simulink library "HMMtoolbox"  (Simulink 8.3)
settings: Solver=ode45  StartTime=0.0  StopTime=10.0  RelTol=1e-3
undefined symbols (not defined in the file): HMMS
libraries: simulink x12
settings Model: Creator=Esrod Zuch  LastModifiedBy=shubo

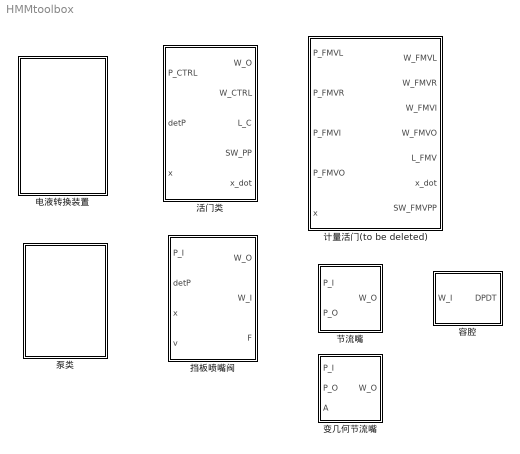
== system HMMtoolbox ==
  变几何节流嘴 : Subsystem  mask{Cqmax=HMMS.JLZ.Cq_max, lamc=1000, rho=HMMS.RHO, nu=HMMS.NU}
      mask prompts: Cqmax "Cq_max(最大流量系数)"; lamc "lamc(临界流数)"; rho "RHO(油液密度kg/m^3)"; nu "NU(油液运动粘度cP)"
  容腔 : Subsystem  mask{B=HMMS.B, V0=HMMS.V(2)}
      mask prompts: B "B(容腔模量kPa)"; V0 "V0(容腔体积m^3)"
  挡板喷嘴阀 : Subsystem  mask{rho=HMMS.RHO, Kv=HMMS.DBPZF.Kv, D_F=HMMS.DBPZF.D_F, D_I=HMMS.DBPZF.D_I, D_R=HMMS.DBPZF.D_R, mode_direct=相反, L_L=0, L_H=HMMS.DBPZF.L_H, x0=HMMS.DBPZF.x0}
      mask prompts: rho "RHO(油液密度kg/m^3)"; Kv "Kv(流量系数)"; D_F "挡板直径(mm)"; D_I "喷嘴内径(mm)"; D_R "杆径(mm)"; mode_direct "开度正方向与阀芯运动正方向"; L_L "L_L(开度低限mm)"; L_H "L_H(开度高限mm)"; x0 "x0(初始遮蔽量mm)"
      mask TypeOptions mode_direct: 相同 | 相反
  泵类 : Subsystem
  活门类 : Subsystem  mask{rho=HMMS.RHO, Kv=HMMS.LJHM.Kv, nu=51, lamc=100, D_P=HMMS.LJHM.D_P, D_R=[0 0], direct_CTRL=[1 -1], mode_direct=相同, L_L=0, L_H=HMMS.LJHM.L_H, m=HMMS.LJHM.m, k=HMMS.LJHM.k, f=HMMS.LJHM.f, f0=HMMS.LJHM.f0, x0=HMMS.LJHM.x0, mode_hole=插值表, C_I=HMMS.LJHM.C_I, C_O=HMMS.LJHM.C_O, D_HOLE=1, n=1}
      mask prompts: rho "RHO(油液密度kg/m^3)"; Kv "Kv_max(最大流量系数)"; nu "NU(油液运动粘度cP)"; lamc "lamc(临界流数)"; D_P "D_P向量(各腔筒径mm)"; D_R "D_R向量(各腔杆径mm)"; direct_CTRL "各腔压力方向向量(推为1拉为-1)"; mode_direct "开度正方向与阀芯运动正方向"; L_L "L_L(位移低限mm)"; L_H "L_H(位移高限mm)"; m "m(阀芯质量kg)"; k "k(弹簧弹性模量N/m)"; f "f(阀芯阻尼N/(m/s))"; f0 "f0(弹簧预紧力N)"; x0 "x0(初始遮蔽量mm)"; mode_hole "计算模式"; C_I "C_I(特性插值输入)"; C_O "C_O(特性插值输出)"; D_HOLE "D_HOLE(圆孔直径mm)"; n "n(圆孔数量)"
      mask TypeOptions mode_direct: 相同 | 相反
      mask TypeOptions mode_hole: 插值表 | 圆面积公式
      mask DialogControl Container13_copy Prompt: 插值表
      mask DialogControl Container13 Prompt: 圆面积公式
  电液转换装置 : Subsystem
  节流嘴 : Subsystem  mask{Cqmax=HMMS.JLZ.Cq_max, lamc=1000, d=HMMS.JLZ.D, rho=HMMS.RHO, nu=HMMS.NU}
      mask prompts: Cqmax "Cq_max(最大流量系数)"; lamc "lamc(临界流数)"; d "D(圆孔直径mm)"; rho "RHO(油液密度kg/m^3)"; nu "NU(油液运动粘度cP)"
  计量活门(to be deleted) : Subsystem  mask(计量活门){L_FMVL=0, L_FMVH=HMMS.HYHM.L_H, D_FMVLP=HMMS.HYHM.D_LP, D_FMVLR=0, D_FMVRP=HMMS.HYHM.D_RP, D_FMVRR=0, C_FMVI=HMMS.HYHM.C_I, C_FMVO=HMMS.HYHM.C_O, f0=HMMS.HYHM.f0, m_FMV=HMMS.HYHM.m, f_FMV=HMMS.HYHM.f, k=HMMS.HYHM.k, rho=HMMS.RHO, Kv_FMV=HMMS.HYHM.Kv}
      mask prompts: L_FMVL "L_FMVL(计量活门位移低限mm)"; L_FMVH "L_FMVH(计量活门位移高限mm)"; D_FMVLP "D_FMVLP(计量活门左腔筒径mm)"; D_FMVLR "D_FMVLR(计量活门左腔杆径mm)"; D_FMVRP "D_FMVRP(计量活门右腔筒径mm)"; D_FMVRR "D_FMVRR(计量活门右腔杆径mm)"; C_FMVI "C_FMVI(计量活门特性插值输入)"; C_FMVO "C_FMVO(计量活门特性插值输出)"; f0 "f0(弹簧预紧力N)"; m_FMV "m_FMV(计量活门阀芯质量kg)"; f_FMV "f_FMV(计量活门阀芯阻尼N/(m/s))"; k "k(计量活门弹簧弹性模量N/m)"; rho "ρ(油液密度kg/m^3)"; Kv_FMV "Kv_FMV(计量活门流量系数)"
      mask help: 填入相关参数

== system HMMtoolbox/变几何节流嘴 ==
  note: Cq
  note: kPa
  note: d/m
  note: m**2/s
  note: Cqmax
  note: m**2
  P_I : Inport
  P_O : Inport  Port=2
  A : Inport  Port=3
  Abs : Abs
  Add : Sum  Inputs=+-
  Constant : Constant  Value=Cqmax
  Constant6 : Constant  Value=nu
  Divide2 : Product  Inputs=*/
  Divide3 : Product  Inputs=**
  Divide4 : Product  Inputs=**
  Fcn : Fcn  Expr=sqrt(2*u*rho)
  Fcn1 : Fcn  Expr=sqrt(4*u/pi)
  Fcn2 : Fcn  Expr=tanh(2*u/lamc)
  Fcn3 : Fcn  Expr=u*1e-3/rho
  Gain1 : Gain  Gain=1e3
  Product : Product
  Product1 : Product  Inputs=3
  Sign : Signum  ZeroCross=off
  W_O : Outport
  wires:
  Sign/1 -> Product/2
  Fcn1/1 -> Divide2/1
  Product/1 -> W_O/1
  Fcn3/1 -> Divide2/2
  Constant6/1 -> Fcn3/1
  Add/1 -> Gain1/1
  Divide4/1 -> Product1/1
  Constant/1 -> Divide4/1
  Fcn2/1 -> Divide4/2
  Divide3/1 -> Fcn2/1
  Divide2/1 -> Divide3/1
  A/1 -> Fcn1/1, Product1/2
  P_I/1 -> Add/1
  Fcn/1 -> Product1/3, Divide3/2
  Abs/1 -> Fcn/1
  Product1/1 -> Product/1
  Gain1/1 -> Abs/1, Sign/1
  P_O/1 -> Add/2

== system HMMtoolbox/容腔 ==
  note: kg
  note: kPa
  note: kg/s
  note: dp/dt kPa/s
  note: V0 m**3
  W_I : Inport
  Constant : Constant  Value=B
  Constant1 : Constant  Value=V0
  Divide : Product  Inputs=**
  Divide1 : Product  Inputs=*/
  Gain1 : Gain  Gain=HMMS.RHO
  Sum of Elements : Sum  Inputs=+
  DPDT : Outport
  wires:
  Divide/1 -> Divide1/1
  Sum of Elements/1 -> Divide/1
  Constant/1 -> Divide/2
  W_I/1 -> Sum of Elements/1
  Divide1/1 -> DPDT/1
  Gain1/1 -> Divide1/2
  Constant1/1 -> Gain1/1

== system HMMtoolbox/挡板喷嘴阀 ==
  P_I : Inport
  detP : Inport  Port=2
  x : Inport  Port=3
  v : Inport  Port=4
  Add1 : Sum
  Add3 : Sum  Inputs=+-
  Gain1 : Gain  Gain=pi*(D_I^2-D_R^2)*10^-3/4
  Gain2 : Gain  Gain=pi*(D_F^2-D_I^2)*10^-3/4
  flowcalc : Subsystem
  W_O : Outport
  W_I : Outport  Port=2
  F : Outport  Port=3
  wires:
  flowcalc/1(W_O) -> W_O/1
  detP/1 -> Add3/2, flowcalc/1(detP)
  x/1 -> flowcalc/2(x)
  flowcalc/2(W_I) -> W_I/1
  v/1 -> flowcalc/3(v)
  P_I/1 -> Gain1/1, Add3/1
  Add3/1 -> Gain2/1
  Gain2/1 -> Add1/2
  Gain1/1 -> Add1/1
  Add1/1 -> F/1

== system HMMtoolbox/泵类 ==
  CLB : Subsystem  mask{mode=平均计算模式, RHO=780, ETA_hym=1, etamode=eta=constant, ETA_V_const=1, ETA_V_tab1=[0 1000 10000], ETA_V_tab2=[1 0.9 0.8], displ=2.2e-7, z1=10, z2=10, m_CLB=2, alpha=20, b_CLB=6}
      mask prompts: mode "齿轮泵计算模式"; RHO "RHO(工质密度kg/m^3)"; ETA_hym "ETA_hym(水力机械效率)"; etamode "计算模式"; ETA_V_const "ETA_V_const(效率常数)"; ETA_V_tab1 "N_tab(转速表rpm)"; ETA_V_tab2 "ETA_V_tab(效率表)"; displ "displ(排量m^3/rad)"; z1 "z1(主动轮齿数(个))"; z2 "z2(从动轮齿数(个))"; m_CLB "m(齿轮模数mm)"; alpha "alpha(齿轮压力角(°))"; b_CLB "b(齿宽mm)"
      mask TypeOptions mode: 平均计算模式 | 脉动计算模式
      mask TypeOptions etamode: eta=constant | eta=f(n)
      mask DialogControl ParameterGroupVar Prompt: 齿轮泵参数设置
      mask DialogControl Container12 Prompt: 模式：eta=constant
      mask DialogControl Container13 Prompt: 模式：eta=f(n)
  LXB : Subsystem  mask{mode=f(qv), ETA=0.8, RHO=780, D=10, D_r=10, N_r=26230, RHO_r=780, W_tab_1=[10000 20000 30000 40000 46400]/780/3600, P_tab_1=[7640	7830	7860	7530	7110], N_tab_2=[18361 19673 20984 22296 23607 24919 26230], W_tab_2=[10000 20000 30000 40000 46400]/780/3600, P_tab_2=[4250,4310,3950,3760,3638.4;4590,4670,4480,4280,4152;5130,5250,5160,4750,4561.76;5680,5830,5740,5400,5200;6280,6430,6400,6050,5700;6970,7150,7140,6800,6430;7640,7830,7860,7530,7110;]}
      mask prompts: mode "mode(计算模式)"; ETA "ETA(泵的工作效率)"; RHO "RHO(实际工质密度(kg/m^3))"; D "D(泵的实际直径mm)"; D_r "D_r(泵的参考直径mm)"; N_r "N_r(泵的参考转速(r/min))"; RHO_r "RHO_r参考工质密度(kg/m^3)"; W_tab_1 "W_tab_1(流量表(m^3/s))"; P_tab_1 "P_tab_1(增压表kPa)"; N_tab_2 "N_tab_2(转速表(r/min))"; W_tab_2 "W_tab_2(流量表m^3/s)"; P_tab_2 "P_tab_2(增压表kPa)"
      mask help: 离心泵模型
      mask TypeOptions mode: f(qv) | f(qv,n)
      mask DialogControl Control2 Prompt: 离心泵模型
  ZSB : Subsystem  mask(柱塞泵){L_ZSBHX=15, D_ZSBZS=48*2, A_ZSBZS=23.8*23.8*pi/4, RHO=780, ETA_V=0.95, Z_ZSBZS=7, BETA_ZSBZS=11/180*pi, A_ZSBTJ=[pi*(33.26^2-17^2)/4, pi*(33.26^2-19.8^2)/4], L_ZSBTJ=[17*2.3/0.6,17*2.48/0.6,42.9,317.743165,165.3], k=((1421-754.6)/((139.7-101.9)-(139.7-119.6))+(1754-1313)/((158-96.8)-(158-114.6)))*1e3, BETA_ZSBSD=7/180*pi, L_x0=30+139.7, J_ZSBXP=0.34, KD=7.65}
      mask prompts: L_ZSBHX "L_HX(等效滑靴厚度mm)"; D_ZSBZS "D_ZS(柱塞轴线在缸体的分布圆直径mm)"; A_ZSBZS "A_ZS(柱塞截面面积mm^2)"; RHO "RHO(标准状态下，油液密度kg/m^3)"; ETA_V "ETA_V(容积效率)"; Z_ZSBZS "Z_ZS(柱塞数量)"; BETA_ZSBZS "BETA_ZS(柱塞安装角rad)"; A_ZSBTJ "A_TJ(面积参数向量mm^2)"; L_ZSBTJ "L_TJ(距离参数向量mm)"; k "k(弹簧弹性模量N/m)"; BETA_ZSBSD "BETA_SD(随动活塞安装角rad)"; L_x0 "L_x0(随动活塞初始位置mm)"; J_ZSBXP "J_XP(斜盘绕斜盘轴的转动惯量kg·m^2)"; KD "KD(斜盘转动阻力系数N·m·s/rad)"
      mask DialogControl DescTextVar Prompt: 填入相关参数

== system HMMtoolbox/活门类 ==
  P_CTRL : Inport
  detP : Inport  Port=2
  x : Inport  Port=3
  Constant4 : Constant  Value=0
  Demux : Demux  Outputs=2
  Gain5 : Gain  Gain=1000
  Mux : Mux  Inputs=2
  Mux1 : Mux  Inputs=2
  flowcalc : Subsystem
  motioncalc : Subsystem
  W_O : Outport
  W_CTRL : Outport  Port=2
  L_C : Outport  Port=3
  SW_PP : Outport  Port=4
  x_dot : Outport  Port=5
  wires:
  motioncalc/4(W_CTRL) -> W_CTRL/1
  flowcalc/1(W_O) -> W_O/1
  detP/1 -> flowcalc/1(detP)
  P_CTRL/1 -> motioncalc/1(P_CTRL)
  Gain5/1 -> L_C/1, flowcalc/2(L_C)
  Demux/2 -> motioncalc/2(v)  "velocity"
  x/1 -> Demux/1
  motioncalc/1(IsMoving) -> Mux1/2
  motioncalc/3(a) -> Mux/2
  Mux1/1 -> SW_PP/1
  Constant4/1 -> Mux1/1
  Demux/1 -> motioncalc/3(x), Gain5/1  "position"
  Mux/1 -> x_dot/1
  motioncalc/2(v_real) -> Mux/1

== system HMMtoolbox/电液转换装置 ==
  HSV23 : Subsystem  mask(电液伺服阀（单个孔特性验证）){Qm=HMMS.HSV23.W_R, delta_Pm=HMMS.HSV23.P_R, Im=HMMS.HSV23.I_R, Wn=HMMS.HSV23.Wn, ksi=HMMS.HSV23.XI, rho=HMMS.RHO}
      mask prompts: Qm "W_R(电液伺服阀额定流量kg/s)"; delta_Pm "P_R(电液伺服阀额定压降kPa)"; Im "I_R(额定电流mA)"; Wn "Wn(阀的自然频率rad/s)"; ksi "ξ(阀的阻尼比)"; rho "ρ(油液密度kg/m^3)"
      mask help: 填入相关参数，和AMESim数据一致
  HSV34 : Subsystem  mask(电液伺服阀（单个孔特性验证）){Qm=HMMS.HSV1.W_R, delta_Pm=HMMS.HSV1.P_R, Im=HMMS.HSV1.I_R, Idet=HMMS.HSV1.I_DELTA, Wn=HMMS.HSV1.Wn, ksi=HMMS.HSV1.XI, rho=HMMS.RHO}
      mask prompts: Qm "W_R(电液伺服阀额定流量kg/s)"; delta_Pm "P_R(电液伺服阀额定压降kPa)"; Im "I_R(额定电流mA)"; Idet "I_DELTA(电流偏置量mA)"; Wn "Wn(阀的自然频率rad/s)"; ksi "ξ(阀的阻尼比)"; rho "ρ(油液密度kg/m^3)"
      mask help: 填入相关参数，和AMESim数据一致

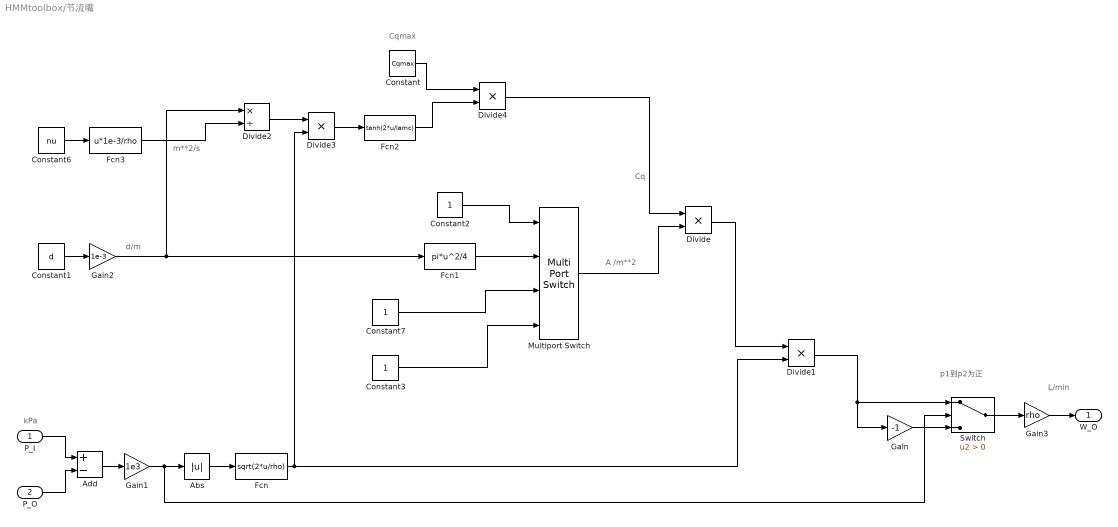
== system HMMtoolbox/节流嘴 ==
  note: L/min
  note: p1到p2为正
  note: Cqmax
  note: m**2/s
  note: d/m
  note: kPa
  note: A /m**2
  note: Cq
  P_I : Inport
  P_O : Inport  Port=2
  Abs : Abs
  Add : Sum  Inputs=+-
  Constant : Constant  Value=Cqmax
  Constant1 : Constant  Value=d
  Constant2 : Constant
  Constant3 : Constant
  Constant6 : Constant  Value=nu
  Constant7 : Constant
  Divide{,1,3..4} (4 alike) : Product  Inputs=**
  Divide2 : Product  Inputs=*/
  Fcn : Fcn  Expr=sqrt(2*u/rho)
  Fcn1 : Fcn  Expr=pi*u^2/4
  Fcn2 : Fcn  Expr=tanh(2*u/lamc)
  Fcn3 : Fcn  Expr=u*1e-3/rho
  Gain : Gain  Gain=-1
  Gain1 : Gain  Gain=1e3
  Gain2 : Gain  Gain=1e-3
  Gain3 : Gain  Gain=rho
  Multiport Switch : MultiPortSwitch
  Switch : Switch  Criteria=u2 > Threshold
  W_O : Outport
  wires:
  P_O/1 -> Add/2
  Gain1/1 -> Switch/2, Abs/1
  Divide1/1 -> Switch/1, Gain/1
  Abs/1 -> Fcn/1
  Fcn/1 -> Divide1/2, Divide3/2
  Divide/1 -> Divide1/1
  P_I/1 -> Add/1
  Gain/1 -> Switch/3
  Multiport Switch/1 -> Divide/2
  Constant2/1 -> Multiport Switch/1
  Fcn1/1 -> Multiport Switch/2
  Constant3/1 -> Multiport Switch/4
  Divide2/1 -> Divide3/1
  Divide3/1 -> Fcn2/1
  Fcn2/1 -> Divide4/2
  Constant/1 -> Divide4/1
  Divide4/1 -> Divide/1
  Add/1 -> Gain1/1
  Constant7/1 -> Multiport Switch/3
  Constant1/1 -> Gain2/1
  Gain2/1 -> Divide2/1, Fcn1/1
  Constant6/1 -> Fcn3/1
  Fcn3/1 -> Divide2/2
  Switch/1 -> Gain3/1
  Gain3/1 -> W_O/1

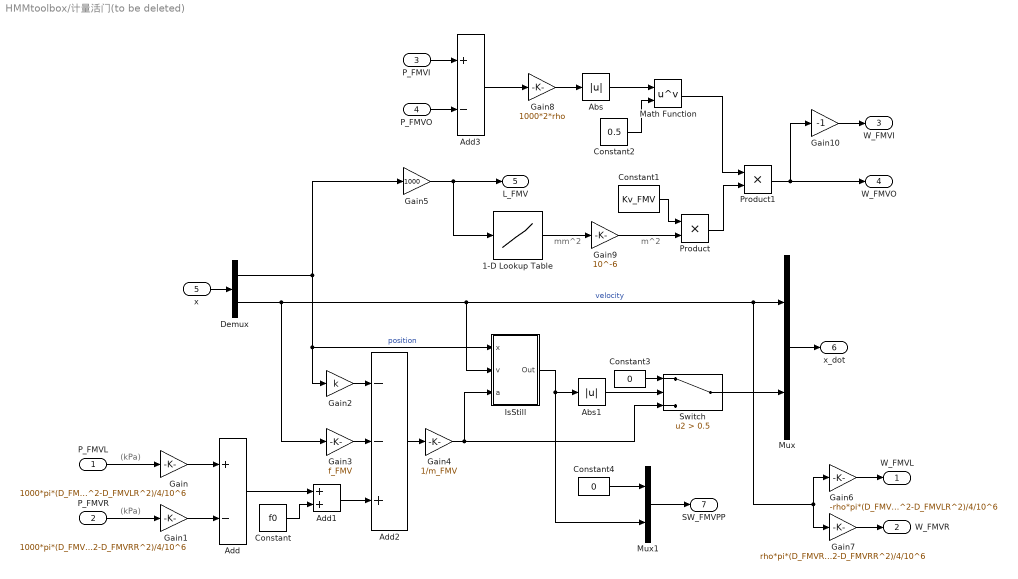
== system HMMtoolbox/计量活门(to be deleted) ==
  note: m^2
  note: mm^2
  note: (kPa)
  note: (kPa)
  P_FMVL : Inport
  P_FMVR : Inport  Port=2
  P_FMVI : Inport  Port=3
  P_FMVO : Inport  Port=4
  x : Inport  Port=5
  1-D Lookup Table : Lookup_n-D  NumberOfTableDimensions=1  BreakpointsForDimension1=C_FMVI  Table=C_FMVO  ExtrapMethod=Clip  UseLastTableValue=on  InternalRulePriority=Speed  RndMeth=Simplest  InputSameDT=on
  Abs : Abs
  Abs1 : Abs
  Add : Sum  Inputs=+-
  Add1 : Sum
  Add2 : Sum  Inputs=--+
  Add3 : Sum  Inputs=+-
  Constant : Constant  Value=f0
  Constant1 : Constant  Value=Kv_FMV
  Constant2 : Constant  Value=0.5
  Constant3 : Constant  Value=0
  Constant4 : Constant  Value=0
  Demux : Demux  Outputs=2
  Gain : Gain  Gain=1000*pi*(D_FMVLP^2-D_FMVLR^2)/4/10^6
  Gain1 : Gain  Gain=1000*pi*(D_FMVRP^2-D_FMVRR^2)/4/10^6
  Gain10 : Gain  Gain=-1
  Gain2 : Gain  Gain=k
  Gain3 : Gain  Gain=f_FMV
  Gain4 : Gain  Gain=1/m_FMV
  Gain5 : Gain  Gain=1000
  Gain6 : Gain  Gain=-rho*pi*(D_FMVLP^2-D_FMVLR^2)/4/10^6
  Gain7 : Gain  Gain=rho*pi*(D_FMVRP^2-D_FMVRR^2)/4/10^6
  Gain8 : Gain  Gain=1000*2*rho
  Gain9 : Gain  Gain=10^-6
  IsStill : Subsystem
  Math Function : Math  Operator=pow  SaturateOnIntegerOverflow=on
  Mux : Mux  Inputs=2
  Mux1 : Mux  Inputs=2
  Product : Product
  Product1 : Product
  Switch : Switch  Criteria=u2 > Threshold  Threshold=0.5
  W_FMVL : Outport
  W_FMVR : Outport  Port=2
  W_FMVI : Outport  Port=3
  W_FMVO : Outport  Port=4
  L_FMV : Outport  Port=5
  x_dot : Outport  Port=6
  SW_FMVPP : Outport  Port=7
  wires:
  Gain5/1 -> 1-D Lookup Table/1, L_FMV/1
  Abs1/1 -> Switch/2
  Demux/2 -> IsStill/2(v), Gain6/1, Gain7/1, Mux/1, Gain3/1  "velocity"
  P_FMVL/1 -> Gain/1
  P_FMVR/1 -> Gain1/1
  x/1 -> Demux/1
  Gain/1 -> Add/1
  Gain7/1 -> W_FMVR/1
  Add3/1 -> Gain8/1
  Product1/1 -> W_FMVO/1, Gain10/1
  Gain10/1 -> W_FMVI/1
  Add/1 -> Add1/1
  Add1/1 -> Add2/3
  Constant/1 -> Add1/2
  Constant2/1 -> Math Function/2
  Gain1/1 -> Add/2
  Gain2/1 -> Add2/1
  Gain3/1 -> Add2/2
  Gain8/1 -> Abs/1
  Abs/1 -> Math Function/1
  Product/1 -> Product1/2
  Gain6/1 -> W_FMVL/1
  1-D Lookup Table/1 -> Gain9/1
  Math Function/1 -> Product1/1
  Constant1/1 -> Product/1
  P_FMVI/1 -> Add3/1
  P_FMVO/1 -> Add3/2
  Add2/1 -> Gain4/1
  Constant3/1 -> Switch/1
  IsStill/1(Out) -> Abs1/1, Mux1/2
  Gain9/1 -> Product/2
  Switch/1 -> Mux/2
  Mux1/1 -> SW_FMVPP/1
  Constant4/1 -> Mux1/1
  Demux/1 -> Gain5/1, Gain2/1, IsStill/1(x)  "position"
  Mux/1 -> x_dot/1
  Gain4/1 -> Switch/3, IsStill/3(a)

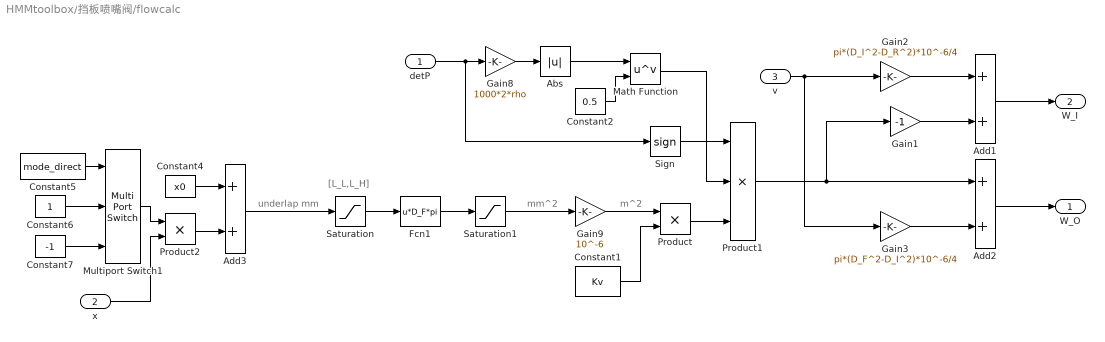
== system HMMtoolbox/挡板喷嘴阀/flowcalc ==
  note: underlap mm
  note: [L_L,L_H]
  note: m^2
  note: mm^2
  detP : Inport
  x : Inport  Port=2
  v : Inport  Port=3
  Abs : Abs
  Add1 : Sum
  Add2 : Sum
  Add3 : Sum
  Constant1 : Constant  Value=Kv
  Constant2 : Constant  Value=0.5
  Constant4 : Constant  Value=x0
  Constant5 : Constant  Value=mode_direct
  Constant6 : Constant
  Constant7 : Constant  Value=-1
  Fcn1 : Fcn  Expr=u*D_F*pi
  Gain1 : Gain  Gain=-1
  Gain2 : Gain  Gain=pi*(D_I^2-D_R^2)*10^-6/4
  Gain3 : Gain  Gain=pi*(D_F^2-D_I^2)*10^-6/4
  Gain8 : Gain  Gain=1000*2*rho
  Gain9 : Gain  Gain=10^-6
  Math Function : Math  Operator=pow  SaturateOnIntegerOverflow=on
  Multiport Switch1 : MultiPortSwitch  Inputs=2
  Product : Product
  Product1 : Product  Inputs=3
  Product2 : Product
  Saturation : Saturate  UpperLimit=L_H  LowerLimit=L_L
  Saturation1 : Saturate  UpperLimit=pi*(D_I^2-D_R^2)/4  LowerLimit=0
  Sign : Signum  ZeroCross=off
  W_O : Outport
  W_I : Outport  Port=2
  wires:
  Multiport Switch1/1 -> Product2/1
  Constant6/1 -> Multiport Switch1/2
  Constant7/1 -> Multiport Switch1/3
  Constant5/1 -> Multiport Switch1/1
  Product2/1 -> Add3/2
  Constant4/1 -> Add3/1
  Saturation1/1 -> Gain9/1
  Fcn1/1 -> Saturation1/1
  Add3/1 -> Saturation/1
  x/1 -> Product2/2
  Math Function/1 -> Product1/2
  Product1/1 -> Add2/1, Gain1/1
  Constant2/1 -> Math Function/2
  Abs/1 -> Math Function/1
  Gain9/1 -> Product/1
  Product/1 -> Product1/3
  Gain8/1 -> Abs/1
  detP/1 -> Gain8/1, Sign/1
  Sign/1 -> Product1/1
  Saturation/1 -> Fcn1/1
  Constant1/1 -> Product/2
  Gain1/1 -> Add1/2
  Add1/1 -> W_I/1
  v/1 -> Gain3/1, Gain2/1
  Gain2/1 -> Add1/1
  Add2/1 -> W_O/1
  Gain3/1 -> Add2/2

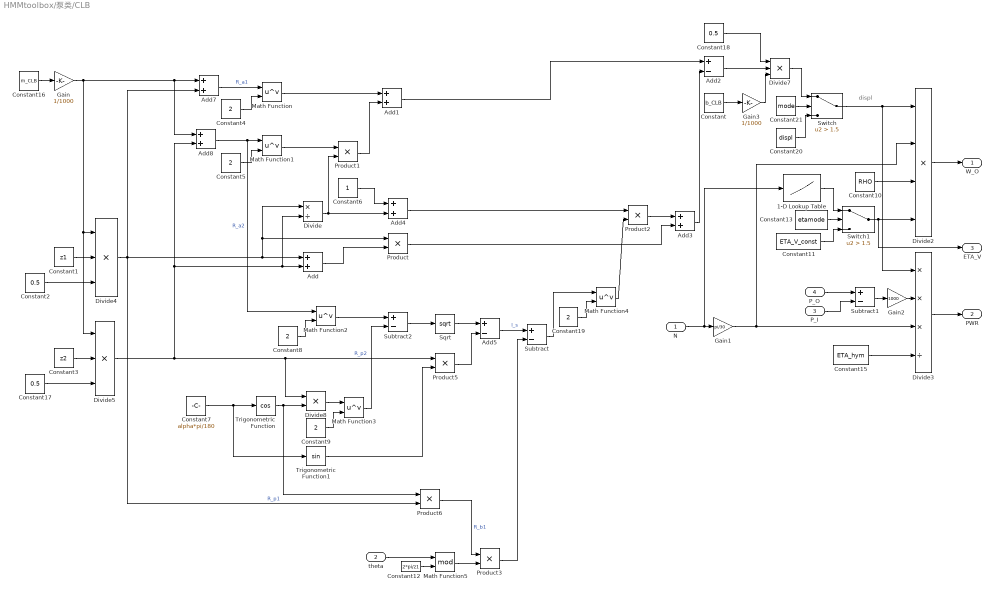
== system HMMtoolbox/泵类/CLB ==
  note: displ
  N : Inport
  theta : Inport  Port=2
  P_I : Inport  Port=3
  P_O : Inport  Port=4
  1-D Lookup Table : Lookup_n-D  NumberOfTableDimensions=1  BreakpointsForDimension1=ETA_V_tab1  Table=ETA_V_tab2  InternalRulePriority=Speed  RndMeth=Simplest  InputSameDT=on
  Add{,1,3..4,7..8} (6 alike) : Sum
  Add2 : Sum  Inputs=+-
  Add5 : Sum  Inputs=+-
  Constant : Constant  Value=b_CLB
  Constant1 : Constant  Value=z1
  Constant10 : Constant  Value=RHO
  Constant11 : Constant  Value=ETA_V_const
  Constant12 : Constant  Value=2*pi/z1
  Constant13 : Constant  Value=etamode
  Constant15 : Constant  Value=ETA_hym
  Constant16 : Constant  Value=m_CLB
  Constant17 : Constant  Value=0.5
  Constant18 : Constant  Value=0.5
  Constant{4..5,8..9,19} (5 alike) : Constant  Value=2
  Constant2 : Constant  Value=0.5
  Constant20 : Constant  Value=displ
  Constant21 : Constant  Value=mode
  Constant3 : Constant  Value=z2
  Constant6 : Constant
  Constant7 : Constant  Value=alpha*pi/180
  Divide : Product  Inputs=*/
  Divide2 : Product  Inputs=****
  Divide3 : Product  Inputs=***/
  Divide4 : Product  Inputs=***
  Divide5 : Product  Inputs=***
  Divide7 : Product  Inputs=***
  Divide8 : Product  Inputs=**
  Gain : Gain  Gain=1/1000
  Gain1 : Gain  Gain=pi/30
  Gain2 : Gain  Gain=1000
  Gain3 : Gain  Gain=1/1000
  Math Function{,1..4} (5 alike) : Math  Operator=pow  SaturateOnIntegerOverflow=on
  Math Function5 : Math  Operator=mod  SaturateOnIntegerOverflow=on
  Product{,1..3,5..6} (6 alike) : Product
  Sqrt : Sqrt  SaturateOnIntegerOverflow=on
  Subtract : Sum  Inputs=+-
  Subtract1 : Sum  Inputs=+-
  Subtract2 : Sum  Inputs=+-
  Switch : Switch  Criteria=u2 > Threshold  Threshold=1.5
  Switch1 : Switch  Criteria=u2 > Threshold  Threshold=1.5
  Trigonometric Function : Trigonometry  Operator=cos
  Trigonometric Function1 : Trigonometry
  W_O : Outport
  PWR : Outport  Port=2
  ETA_V : Outport  Port=3
  wires:
  P_I/1 -> Subtract1/2
  P_O/1 -> Subtract1/1
  Math Function1/1 -> Product1/1
  Product1/1 -> Add1/2
  Add4/1 -> Product2/1
  Product/1 -> Add3/2
  Add3/1 -> Add2/2
  Add8/1 -> Math Function1/1, Math Function2/1  "R_a2"
  Constant4/1 -> Math Function/2
  Divide4/1 -> Product6/2, Product/1, Divide/1, Add/1, Add7/2  "R_p1"
  Add/1 -> Product/2
  Math Function/1 -> Add1/1
  Add7/1 -> Math Function/1  "R_a1"
  Constant5/1 -> Math Function1/2
  Divide/1 -> Add4/2, Product1/2
  Constant6/1 -> Add4/1
  Add1/1 -> Add2/1
  Product2/1 -> Add3/1
  Divide5/1 -> Product5/1, Divide8/1, Add/2, Divide/2, Add8/2  "R_p2"
  Add5/1 -> Subtract/1  "l_s"
  Subtract/1 -> Math Function4/1
  Subtract2/1 -> Sqrt/1
  Sqrt/1 -> Add5/1
  Constant9/1 -> Math Function3/2
  Trigonometric Function1/1 -> Product5/2
  Constant8/1 -> Math Function2/2
  Constant7/1 -> Trigonometric Function/1, Trigonometric Function1/1
  Product5/1 -> Add5/2
  Math Function2/1 -> Subtract2/1
  Divide2/1 -> W_O/1
  Divide3/1 -> PWR/1
  Constant16/1 -> Gain/1
  Constant1/1 -> Divide4/2
  Constant2/1 -> Divide4/3
  Constant3/1 -> Divide5/2
  Constant17/1 -> Divide5/3
  Add2/1 -> Divide7/2
  Constant18/1 -> Divide7/1
  Gain/1 -> Divide5/1, Divide4/1, Add7/1, Add8/1
  Math Function3/1 -> Subtract2/2
  Divide8/1 -> Math Function3/1
  Trigonometric Function/1 -> Product6/1, Divide8/2
  Product6/1 -> Product3/1  "R_b1"
  Product3/1 -> Subtract/2
  Gain2/1 -> Divide3/2
  Subtract1/1 -> Gain2/1
  Constant19/1 -> Math Function4/2
  Math Function4/1 -> Product2/2
  Constant/1 -> Gain3/1
  Gain3/1 -> Divide7/3
  Constant10/1 -> Divide2/3
  Constant21/1 -> Switch/2
  Switch/1 -> Divide3/1, Divide2/1
  Constant15/1 -> Divide3/4
  Constant20/1 -> Switch/3
  Divide7/1 -> Switch/1
  N/1 -> 1-D Lookup Table/1, Gain1/1
  Gain1/1 -> Divide2/2, Divide3/3
  theta/1 -> Math Function5/1
  Math Function5/1 -> Product3/2
  Constant12/1 -> Math Function5/2
  Constant13/1 -> Switch1/2
  Switch1/1 -> ETA_V/1, Divide2/4
  Constant11/1 -> Switch1/3
  1-D Lookup Table/1 -> Switch1/1

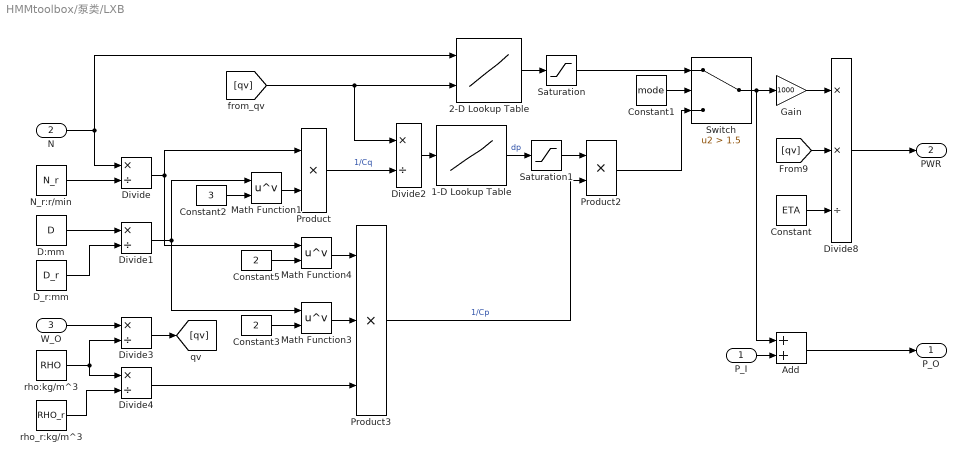
== system HMMtoolbox/泵类/LXB ==
  "\tP_I" : Inport
  N : Inport  Port=2
  W_O : Inport  Port=3
  1-D Lookup Table : Lookup_n-D  NumberOfTableDimensions=1  BreakpointsForDimension1=W_tab_1  Table=P_tab_1  InternalRulePriority=Speed  RndMeth=Simplest  InputSameDT=on
  2-D Lookup Table : Lookup_n-D  BreakpointsForDimension1=N_tab_2  BreakpointsForDimension2=W_tab_2  Table=P_tab_2  InternalRulePriority=Speed  RndMeth=Simplest  InputSameDT=on
  Add : Sum
  Constant : Constant  Value=ETA
  Constant1 : Constant  Value=mode
  Constant2 : Constant  Value=3
  Constant3 : Constant  Value=2
  Constant5 : Constant  Value=2
  D:mm : Constant  Value=D
  D_r:mm : Constant  Value=D_r
  Divide{,1..4} (5 alike) : Product  Inputs=*/
  Divide8 : Product  Inputs=**/
  Gain : Gain  Gain=1000
  Math Function1 : Math  Operator=pow  SaturateOnIntegerOverflow=on
  Math Function3 : Math  Operator=pow  SaturateOnIntegerOverflow=on
  Math Function4 : Math  Operator=pow  SaturateOnIntegerOverflow=on
  N_r:r/min : Constant  Value=N_r
  Product : Product
  Product2 : Product
  Product3 : Product  Inputs=3
  Saturation : Saturate  UpperLimit=inf  LowerLimit=0
  Saturation1 : Saturate  UpperLimit=inf  LowerLimit=0
  Switch : Switch  Criteria=u2 > Threshold  Threshold=1.5
  rho:kg/m^3 : Constant  Value=RHO
  rho_r:kg/m^3 : Constant  Value=RHO_r
  P_O : Outport
  PWR : Outport  Port=2
  wires:
  Add/1 -> P_O/1
  N_r:r/min/1 -> Divide/2
  D:mm/1 -> Divide1/1
  D_r:mm/1 -> Divide1/2
  rho:kg/m^3/1 -> Divide4/1, Divide3/2
  rho_r:kg/m^3/1 -> Divide4/2
  Constant2/1 -> Math Function1/2
  Constant5/1 -> Math Function4/2
  Constant3/1 -> Math Function3/2
  Divide1/1 -> Math Function3/1, Math Function1/1
  Math Function4/1 -> Product3/1
  Math Function3/1 -> Product3/2
  Divide4/1 -> Product3/3
  Math Function1/1 -> Product/2
  Product/1 -> Divide2/2  "1/Cq"
  Divide2/1 -> 1-D Lookup Table/1
  Divide3/1 -> [qv]
  Constant/1 -> Divide8/3
  [qv] -> Divide8/2
  Switch/1 -> Add/1, Gain/1
  Divide8/1 -> PWR/1
  Constant1/1 -> Switch/2
  Product3/1 -> Product2/2  "1/Cp"
  W_O/1 -> Divide3/1
  N/1 -> Divide/1, 2-D Lookup Table/1
  Gain/1 -> Divide8/1
  Divide/1 -> Math Function4/1, Product/1
  Product2/1 -> Switch/3
  "\tP_I"/1 -> Add/2
  2-D Lookup Table/1 -> Saturation/1
  1-D Lookup Table/1 -> Saturation1/1  "dp"
  Saturation1/1 -> Product2/1
  [qv] -> Divide2/1, 2-D Lookup Table/2
  Saturation/1 -> Switch/1

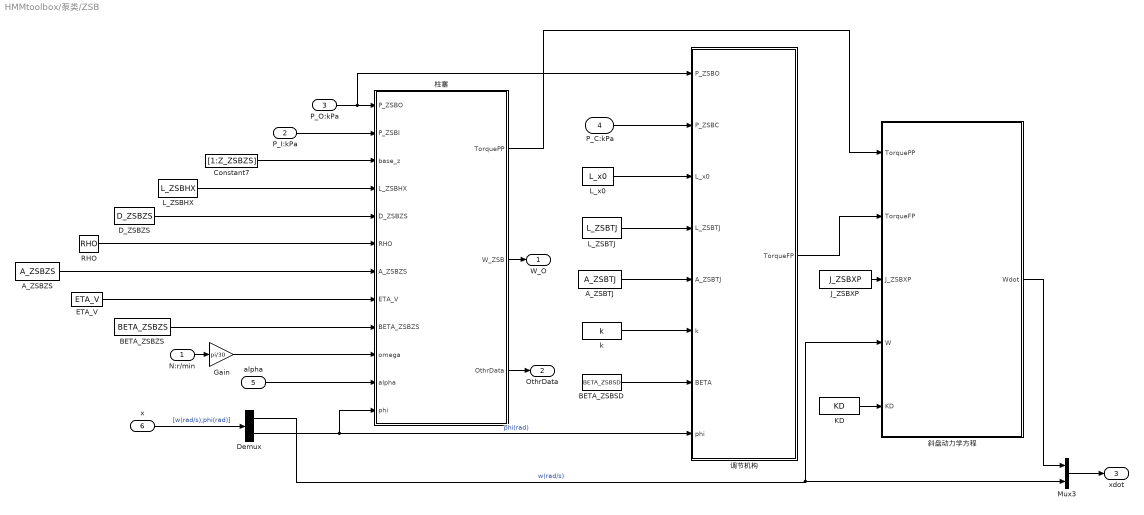
== system HMMtoolbox/泵类/ZSB ==
  N:r/min : Inport
  P_I:kPa : Inport  Port=2
  P_O:kPa : Inport  Port=3
  P_C:kPa : Inport  Port=4
  alpha : Inport  Port=5
  x : Inport  Port=6
  A_ZSBTJ : Constant  Value=A_ZSBTJ
  A_ZSBZS : Constant  Value=A_ZSBZS
  BETA_ZSBSD : Constant  Value=BETA_ZSBSD
  BETA_ZSBZS : Constant  Value=BETA_ZSBZS
  Constant7 : Constant  Value=[1:Z_ZSBZS]
  D_ZSBZS : Constant  Value=D_ZSBZS
  Demux : Demux  Outputs=2
  ETA_V : Constant  Value=ETA_V
  Gain : Gain  Gain=pi/30
  J_ZSBXP : Constant  Value=J_ZSBXP
  KD : Constant  Value=KD
  L_ZSBHX : Constant  Value=L_ZSBHX
  L_ZSBTJ : Constant  Value=L_ZSBTJ
  L_x0 : Constant  Value=L_x0
  Mux3 : Mux  Inputs=2
  RHO : Constant  Value=RHO
  k : Constant  Value=k
  斜盘动力学方程 : MATLAB Function  TreatAsAtomicUnit=on
  柱塞 : MATLAB Function  TreatAsAtomicUnit=on
  调节机构 : MATLAB Function  TreatAsAtomicUnit=on
  W_O : Outport
  OthrData : Outport  Port=2
  xdot : Outport  Port=3
  wires:
  KD/1 -> 斜盘动力学方程/5(KD)
  调节机构/1(TorqueFP) -> 斜盘动力学方程/2(TorqueFP)
  P_I:kPa/1 -> 柱塞/2(P_ZSBI)
  P_C:kPa/1 -> 调节机构/2(P_ZSBC)
  Demux/2 -> 柱塞/12(phi), 调节机构/8(phi)  "phi(rad)"
  N:r/min/1 -> Gain/1
  A_ZSBZS/1 -> 柱塞/7(A_ZSBZS)
  Constant7/1 -> 柱塞/3(base_z)
  RHO/1 -> 柱塞/6(RHO)
  L_ZSBHX/1 -> 柱塞/4(L_ZSBHX)
  L_ZSBTJ/1 -> 调节机构/4(L_ZSBTJ)
  P_O:kPa/1 -> 调节机构/1(P_ZSBO), 柱塞/1(P_ZSBO)
  BETA_ZSBSD/1 -> 调节机构/7(BETA)
  Gain/1 -> 柱塞/10(omega)
  L_x0/1 -> 调节机构/3(L_x0)
  柱塞/1(TorquePP) -> 斜盘动力学方程/1(TorquePP)
  k/1 -> 调节机构/6(k)
  柱塞/2(W_ZSB) -> W_O/1
  Demux/1 -> Mux3/2, 斜盘动力学方程/4(W)  "w(rad/s)"
  D_ZSBZS/1 -> 柱塞/5(D_ZSBZS)
  ETA_V/1 -> 柱塞/8(ETA_V)
  BETA_ZSBZS/1 -> 柱塞/9(BETA_ZSBZS)
  A_ZSBTJ/1 -> 调节机构/5(A_ZSBTJ)
  J_ZSBXP/1 -> 斜盘动力学方程/3(J_ZSBXP)
  alpha/1 -> 柱塞/11(alpha)
  柱塞/3(OthrData) -> OthrData/1
  Mux3/1 -> xdot/1
  斜盘动力学方程/1(Wdot) -> Mux3/1
  x/1 -> Demux/1  "[w(rad/s);phi(rad)]"

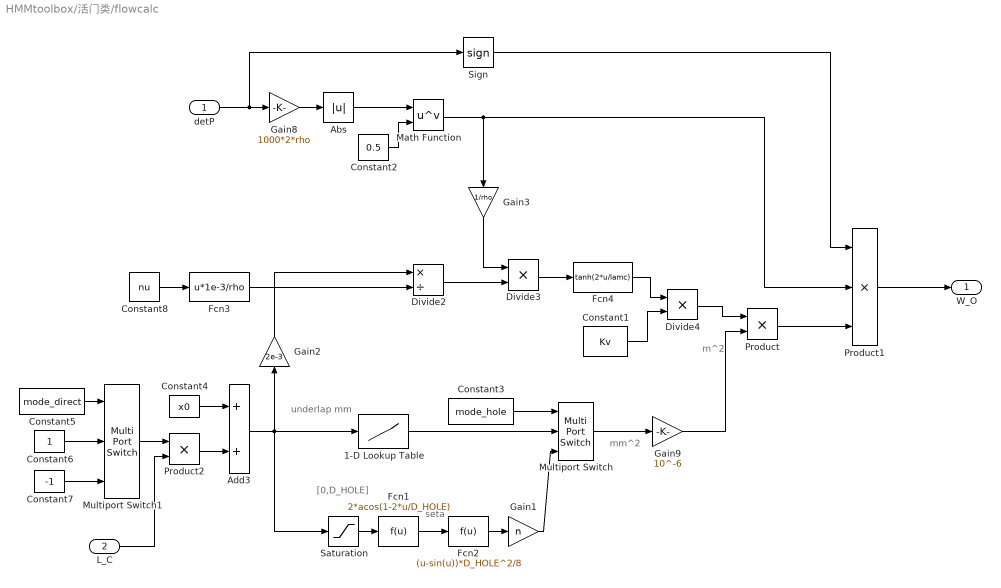
== system HMMtoolbox/活门类/flowcalc ==
  note: underlap mm
  note: seta
  note: [0,D_HOLE]
  note: m^2
  note: mm^2
  detP : Inport
  L_C : Inport  Port=2
  1-D Lookup Table : Lookup_n-D  NumberOfTableDimensions=1  BreakpointsForDimension1=C_I  Table=C_O  ExtrapMethod=Clip  UseLastTableValue=on  InternalRulePriority=Speed  RndMeth=Simplest  InputSameDT=on
  Abs : Abs
  Add3 : Sum
  Constant1 : Constant  Value=Kv
  Constant2 : Constant  Value=0.5
  Constant3 : Constant  Value=mode_hole
  Constant4 : Constant  Value=x0
  Constant5 : Constant  Value=mode_direct
  Constant6 : Constant
  Constant7 : Constant  Value=-1
  Constant8 : Constant  Value=nu
  Divide2 : Product  Inputs=*/
  Divide3 : Product  Inputs=**
  Divide4 : Product  Inputs=**
  Fcn1 : Fcn  Expr=2*acos(1-2*u/D_HOLE)
  Fcn2 : Fcn  Expr=(u-sin(u))*D_HOLE^2/8
  Fcn3 : Fcn  Expr=u*1e-3/rho
  Fcn4 : Fcn  Expr=tanh(2*u/lamc)
  Gain1 : Gain  Gain=n
  Gain2 : Gain  Gain=2e-3
  Gain3 : Gain  Gain=1/rho
  Gain8 : Gain  Gain=1000*2*rho
  Gain9 : Gain  Gain=10^-6
  Math Function : Math  Operator=pow  SaturateOnIntegerOverflow=on
  Multiport Switch : MultiPortSwitch  Inputs=2
  Multiport Switch1 : MultiPortSwitch  Inputs=2
  Product : Product
  Product1 : Product  Inputs=3
  Product2 : Product
  Saturation : Saturate  UpperLimit=D_HOLE  LowerLimit=0
  Sign : Signum  ZeroCross=off
  W_O : Outport
  wires:
  Multiport Switch1/1 -> Product2/1
  Constant6/1 -> Multiport Switch1/2
  Constant7/1 -> Multiport Switch1/3
  Constant5/1 -> Multiport Switch1/1
  Product2/1 -> Add3/2
  Constant4/1 -> Add3/1
  1-D Lookup Table/1 -> Multiport Switch/2
  Gain1/1 -> Multiport Switch/3
  Multiport Switch/1 -> Gain9/1
  Fcn2/1 -> Gain1/1
  Fcn1/1 -> Fcn2/1
  Add3/1 -> 1-D Lookup Table/1, Saturation/1, Gain2/1
  L_C/1 -> Product2/2
  Saturation/1 -> Fcn1/1
  Constant3/1 -> Multiport Switch/1
  Product1/1 -> W_O/1
  Constant2/1 -> Math Function/2
  Abs/1 -> Math Function/1
  Gain9/1 -> Product/2
  Gain8/1 -> Abs/1
  detP/1 -> Gain8/1, Sign/1
  Constant8/1 -> Fcn3/1
  Fcn3/1 -> Divide2/2
  Gain2/1 -> Divide2/1
  Divide2/1 -> Divide3/2
  Math Function/1 -> Product1/2, Gain3/1
  Gain3/1 -> Divide3/1
  Divide3/1 -> Fcn4/1
  Divide4/1 -> Product/1
  Constant1/1 -> Divide4/2
  Fcn4/1 -> Divide4/1
  Sign/1 -> Product1/1
  Product/1 -> Product1/3

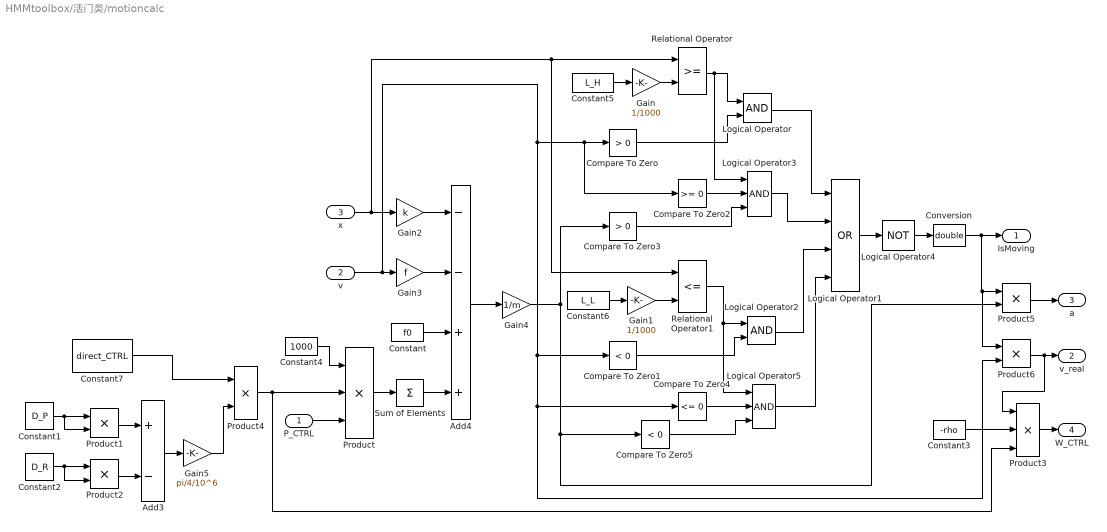
== system HMMtoolbox/活门类/motioncalc ==
  P_CTRL : Inport
  v : Inport  Port=2
  x : Inport  Port=3
  Add3 : Sum  Inputs=+-
  Add4 : Sum  Inputs=--++
  Compare To Zero : simulink/Logic and Bit Operations/Compare To Zero  relop=>  OutDataTypeStr=boolean  ZeroCross=off
  Compare To Zero1 : simulink/Logic and Bit Operations/Compare To Zero  relop=<  OutDataTypeStr=boolean  ZeroCross=off
  Compare To Zero2 : simulink/Logic and Bit Operations/Compare To Zero  relop=>=  OutDataTypeStr=boolean
  Compare To Zero3 : simulink/Logic and Bit Operations/Compare To Zero  relop=>  OutDataTypeStr=boolean
  Compare To Zero4 : simulink/Logic and Bit Operations/Compare To Zero  relop=<=  OutDataTypeStr=boolean  ZeroCross=off
  Compare To Zero5 : simulink/Logic and Bit Operations/Compare To Zero  relop=<  OutDataTypeStr=boolean
  Constant : Constant  Value=f0
  Constant1 : Constant  Value=D_P
  Constant2 : Constant  Value=D_R
  Constant3 : Constant  Value=-rho
  Constant4 : Constant  Value=1000
  Constant5 : Constant  Value=L_H
  Constant6 : Constant  Value=L_L
  Constant7 : Constant  Value=direct_CTRL
  Conversion : DataTypeConversion  OutDataTypeStr=double
  Gain : Gain  Gain=1/1000
  Gain1 : Gain  Gain=1/1000
  Gain2 : Gain  Gain=k
  Gain3 : Gain  Gain=f
  Gain4 : Gain  Gain=1/m
  Gain5 : Gain  Gain=pi/4/10^6
  Logical Operator : Logic  AllPortsSameDT=off  OutDataTypeStr=boolean
  Logical Operator1 : Logic  Operator=OR  Inputs=4  AllPortsSameDT=off  OutDataTypeStr=boolean
  Logical Operator2 : Logic  AllPortsSameDT=off  OutDataTypeStr=boolean
  Logical Operator3 : Logic  Inputs=3  AllPortsSameDT=off  OutDataTypeStr=boolean
  Logical Operator4 : Logic  Operator=NOT  Inputs=4  AllPortsSameDT=off  OutDataTypeStr=boolean
  Logical Operator5 : Logic  Inputs=3  AllPortsSameDT=off  OutDataTypeStr=boolean
  Product : Product  Inputs=3
  Product{1..2,4..6} (5 alike) : Product
  Product3 : Product  Inputs=3
  Relational Operator : RelationalOperator  OutDataTypeStr=boolean
  Relational Operator1 : RelationalOperator  Operator=<=  OutDataTypeStr=boolean  ZeroCross=off
  Sum of Elements : Sum  Inputs=+
  IsMoving : Outport
  v_real : Outport  Port=2
  a : Outport  Port=3
  W_CTRL : Outport  Port=4
  wires:
  Product4/1 -> Product3/3, Product/2
  Gain5/1 -> Product4/2
  Constant7/1 -> Product4/1
  Constant4/1 -> Product/1
  Product3/1 -> W_CTRL/1
  Conversion/1 -> Product6/1, Product5/1, IsMoving/1
  Logical Operator1/1 -> Logical Operator4/1
  Logical Operator5/1 -> Logical Operator1/4
  Logical Operator2/1 -> Logical Operator1/3
  Constant2/1 -> Product2/1, Product2/2
  Gain2/1 -> Add4/1
  Logical Operator/1 -> Logical Operator1/1
  Compare To Zero3/1 -> Logical Operator3/3
  Compare To Zero2/1 -> Logical Operator3/2
  Compare To Zero1/1 -> Logical Operator2/2
  Relational Operator/1 -> Logical Operator/1, Logical Operator3/1
  Constant5/1 -> Gain/1
  v/1 -> Gain3/1, Compare To Zero/1, Compare To Zero2/1, Compare To Zero1/1, Product6/2, Compare To Zero4/1
  Constant6/1 -> Gain1/1
  Compare To Zero/1 -> Logical Operator/2
  x/1 -> Relational Operator/1, Relational Operator1/1, Gain2/1
  Gain/1 -> Relational Operator/2
  Compare To Zero4/1 -> Logical Operator5/2
  Gain4/1 -> Product5/2, Compare To Zero5/1, Compare To Zero3/1
  Logical Operator3/1 -> Logical Operator1/2
  Compare To Zero5/1 -> Logical Operator5/3
  Relational Operator1/1 -> Logical Operator2/1, Logical Operator5/1
  Gain1/1 -> Relational Operator1/2
  Gain3/1 -> Add4/2
  Constant1/1 -> Product1/2, Product1/1
  Product2/1 -> Add3/2
  Constant/1 -> Add4/3
  Product1/1 -> Add3/1
  Product/1 -> Sum of Elements/1
  Add4/1 -> Gain4/1
  Logical Operator4/1 -> Conversion/1
  Add3/1 -> Gain5/1
  P_CTRL/1 -> Product/3
  Sum of Elements/1 -> Add4/4
  Product5/1 -> a/1
  Product6/1 -> Product3/1, v_real/1
  Constant3/1 -> Product3/2

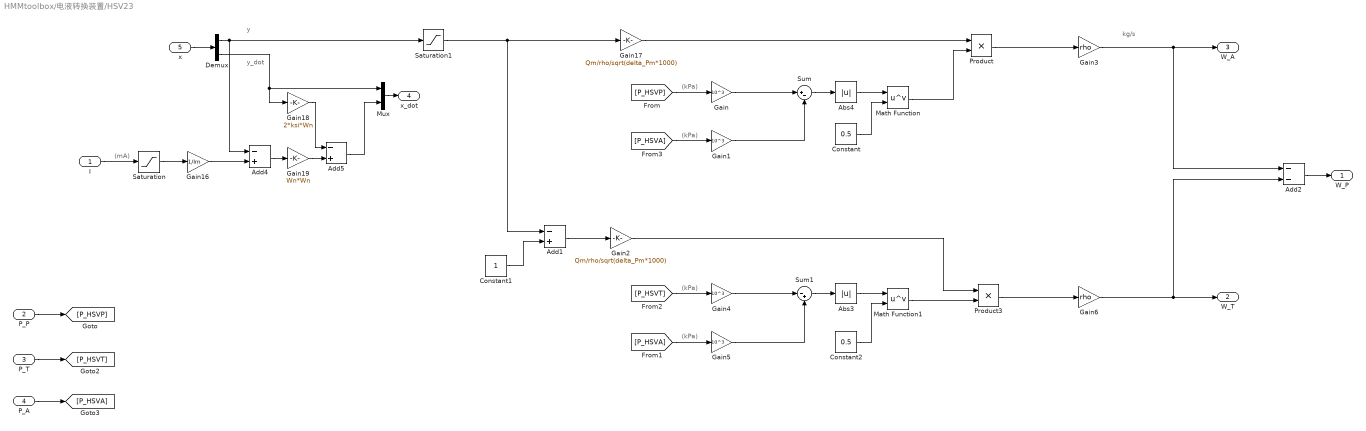
== system HMMtoolbox/电液转换装置/HSV23 ==
  note: (kPa)
  note: (kPa)
  note: (mA)
  note: (kPa)
  note: (kPa)
  note: kg/s
  note: y
  note: y_dot
  I : Inport
  P_P : Inport  Port=2
  P_T : Inport  Port=3
  P_A : Inport  Port=4
  x : Inport  Port=5
  Abs3 : Abs
  Abs4 : Abs
  Add1 : Sum  Inputs=-+
  Add2 : Sum  Inputs=--
  Add4 : Sum  Inputs=-+
  Add5 : Sum  Inputs=-+
  Constant : Constant  Value=0.5
  Constant1 : Constant
  Constant2 : Constant  Value=0.5
  Demux : Demux  Outputs=2
  Gain{,1,4..5} (4 alike) : Gain  Gain=10^3
  Gain16 : Gain  Gain=1/Im
  Gain17 : Gain  Gain=Qm/rho/sqrt(delta_Pm*1000)
  Gain18 : Gain  Gain=2*ksi*Wn
  Gain19 : Gain  Gain=Wn*Wn
  Gain2 : Gain  Gain=Qm/rho/sqrt(delta_Pm*1000)
  Gain3 : Gain  Gain=rho
  Gain6 : Gain  Gain=rho
  Math Function : Math  Operator=pow  SaturateOnIntegerOverflow=on
  Math Function1 : Math  Operator=pow  SaturateOnIntegerOverflow=on
  Mux : Mux  Inputs=2
  Product : Product
  Product3 : Product
  Saturation : Saturate  UpperLimit=Im  LowerLimit=0
  Saturation1 : Saturate  UpperLimit=1  LowerLimit=0
  Sum : Sum  Inputs=|+-
  Sum1 : Sum  Inputs=|-+
  W_P : Outport
  W_T : Outport  Port=2
  W_A : Outport  Port=3
  x_dot : Outport  Port=4
  wires:
  Mux/1 -> x_dot/1
  Add5/1 -> Mux/2
  Gain18/1 -> Add5/1
  Gain19/1 -> Add5/2
  Add4/1 -> Gain19/1
  Gain16/1 -> Add4/2
  Demux/2 -> Gain18/1, Mux/1
  x/1 -> Demux/1
  Gain17/1 -> Product/1
  Abs4/1 -> Math Function/1
  Abs3/1 -> Math Function1/1
  Product3/1 -> Gain6/1
  Product/1 -> Gain3/1
  Gain3/1 -> W_A/1, Add2/1
  Add2/1 -> W_P/1
  Gain6/1 -> Add2/2, W_T/1
  [P_HSVA] -> Gain5/1
  [P_HSVT] -> Gain4/1
  [P_HSVA] -> Gain1/1
  [P_HSVP] -> Gain/1
  P_T/1 -> [P_HSVT]
  P_A/1 -> [P_HSVA]
  P_P/1 -> [P_HSVP]
  Math Function1/1 -> Product3/2
  Gain5/1 -> Sum1/2
  Gain4/1 -> Sum1/1
  Constant2/1 -> Math Function1/2
  Sum1/1 -> Abs3/1
  Gain1/1 -> Sum/2
  Gain/1 -> Sum/1
  Saturation/1 -> Gain16/1
  Constant/1 -> Math Function/2
  Sum/1 -> Abs4/1
  I/1 -> Saturation/1
  Math Function/1 -> Product/2
  Demux/1 -> Saturation1/1, Add4/1
  Saturation1/1 -> Add1/1, Gain17/1
  Add1/1 -> Gain2/1
  Gain2/1 -> Product3/1
  Constant1/1 -> Add1/2

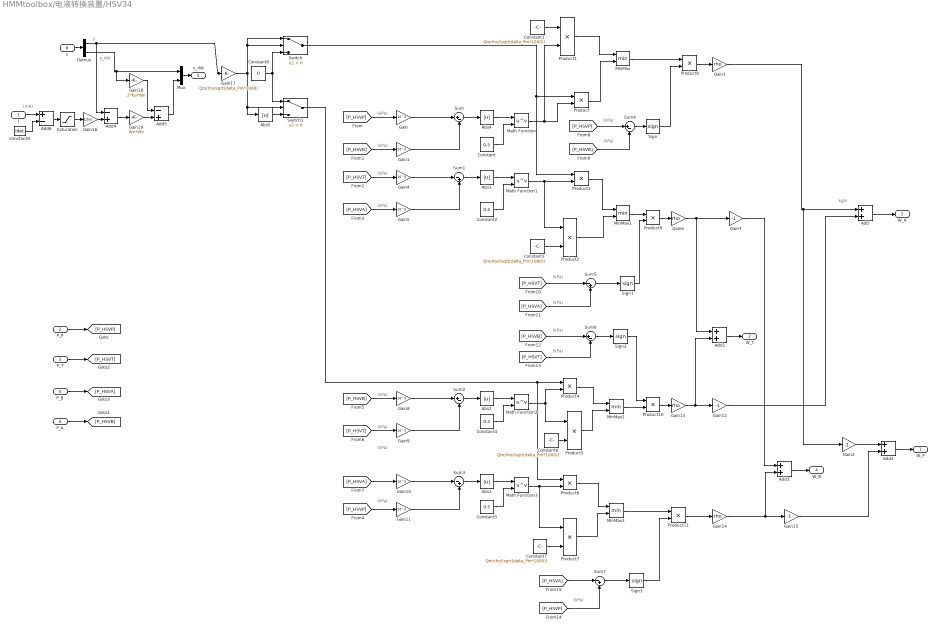
== system HMMtoolbox/电液转换装置/HSV34 ==
  note: y_dot
  note: y
  note: kg/s
  note: (kPa)
  note: (kPa)
  note: (mA)
  note: (kPa)
  note: (kPa)
  note: (kPa)
  note: (kPa)
  note: (kPa)
  note: (kPa)
  note: (kPa)
  note: (kPa)
  note: (kPa)
  note: (kPa)
  note: (kPa)
  note: (kPa)
  note: (kPa)
  I : Inport
  P_P : Inport  Port=2
  P_T : Inport  Port=3
  P_A : Inport  Port=4
  P_B : Inport  Port=5
  x : Inport  Port=6
  Abs{1..5} (5 alike) : Abs
  Add{,1..3} (4 alike) : Sum
  Add4 : Sum  Inputs=-+
  Add5 : Sum  Inputs=-+
  Add6 : Sum  Inputs=+-
  Constant{,2,4..5} (4 alike) : Constant  Value=0.5
  Constant{1,3,6..7} (4 alike) : Constant  Value=Qm/rho/(sqrt(delta_Pm*1000))
  Constant8 : Constant  Value=0
  Constant9 : Constant  Value=Idet
  Demux : Demux  Outputs=2
  Gain{,1,4..5,8..11} (8 alike) : Gain  Gain=10^3
  Gain{2,7,12,15} (4 alike) : Gain  Gain=-1
  Gain{3,6,13..14} (4 alike) : Gain  Gain=rho
  Gain16 : Gain  Gain=1/Im
  Gain17 : Gain  Gain=Qm/rho/sqrt(delta_Pm*1000)
  Gain18 : Gain  Gain=2*ksi*Wn
  Gain19 : Gain  Gain=Wn*Wn
  Math Function{,1..3} (4 alike) : Math  Operator=pow  SaturateOnIntegerOverflow=on
  MinMax{,1..3} (4 alike) : MinMax  Inputs=2
  Mux : Mux  Inputs=2
  Product{,1..11} (12 alike) : Product
  Saturation : Saturate  UpperLimit=Im  LowerLimit=-Im
  Sign{,1..3} (4 alike) : Signum
  Sum{,2,4,6} (4 alike) : Sum  Inputs=|+-
  Sum{1,3,5,7} (4 alike) : Sum  Inputs=|-+
  Switch : Switch  Criteria=u2 > Threshold
  Switch1 : Switch  Criteria=u2 > Threshold
  W_P : Outport
  W_T : Outport  Port=2
  W_A : Outport  Port=3
  W_B : Outport  Port=4
  x_dot : Outport  Port=5
  wires:
  Constant9/1 -> Add6/2
  Sign/1 -> Product8/2
  MinMax/1 -> Product8/1
  Add6/1 -> Saturation/1
  Math Function/1 -> Product1/2, Product/2
  I/1 -> Add6/1
  Sum/1 -> Abs4/1
  Constant/1 -> Math Function/2
  Product/1 -> MinMax/2
  Constant1/1 -> Product1/1
  Product1/1 -> MinMax/1
  Saturation/1 -> Gain16/1
  Gain/1 -> Sum/1
  Gain1/1 -> Sum/2
  Gain3/1 -> Gain2/1, Add/1
  Sum1/1 -> Abs3/1
  Constant2/1 -> Math Function1/2
  Gain4/1 -> Sum1/1
  Gain5/1 -> Sum1/2
  Constant3/1 -> Product2/2
  Math Function1/1 -> Product2/1, Product3/2
  Product3/1 -> MinMax1/1
  Product2/1 -> MinMax1/2
  Gain6/1 -> Add1/1, Gain7/1
  Gain7/1 -> Add3/1
  Sum2/1 -> Abs2/1
  [P_HSVB] -> Gain8/1
  Constant4/1 -> Math Function2/2
  Gain8/1 -> Sum2/1
  Gain9/1 -> Sum2/2
  Sum3/1 -> Abs1/1
  [P_HSVP] -> Gain11/1
  Constant5/1 -> Math Function3/2
  Gain10/1 -> Sum3/1
  Gain11/1 -> Sum3/2
  P_P/1 -> [P_HSVP]
  P_A/1 -> [P_HSVB]
  P_T/1 -> [P_HSVT]
  P_B/1 -> [P_HSVA]
  [P_HSVP] -> Gain/1
  [P_HSVB] -> Gain1/1
  [P_HSVT] -> Gain4/1
  [P_HSVA] -> Gain5/1
  [P_HSVT] -> Gain9/1
  [P_HSVA] -> Gain10/1
  Switch1/1 -> Product6/1, Product4/1
  Math Function2/1 -> Product5/1, Product4/2
  Constant6/1 -> Product5/2
  Product4/1 -> MinMax2/1
  Product5/1 -> MinMax2/2
  Gain13/1 -> Add1/2, Gain12/1
  Add/1 -> W_A/1
  Gain12/1 -> Add/2
  Add1/1 -> W_T/1
  Math Function3/1 -> Product7/1, Product6/2
  Constant7/1 -> Product7/2
  Product6/1 -> MinMax3/1
  Product7/1 -> MinMax3/2
  Gain14/1 -> Add3/2, Gain15/1
  Add2/1 -> W_P/1
  Gain2/1 -> Add2/1
  Gain15/1 -> Add2/2
  Add3/1 -> W_B/1
  Sum4/1 -> Sign/1
  Sum5/1 -> Sign1/1
  [P_HSVT] -> Sum5/1
  [P_HSVA] -> Sum5/2
  [P_HSVP] -> Sum4/1
  [P_HSVB] -> Sum4/2
  Product8/1 -> Gain3/1
  MinMax1/1 -> Product9/1
  Product9/1 -> Gain6/1
  Sign1/1 -> Product9/2
  Sum6/1 -> Sign2/1
  [P_HSVB] -> Sum6/1
  [P_HSVT] -> Sum6/2
  MinMax2/1 -> Product10/2
  Product10/1 -> Gain13/1
  Sign2/1 -> Product10/1
  [P_HSVA] -> Sum7/1
  [P_HSVP] -> Sum7/2
  Sum7/1 -> Sign3/1
  MinMax3/1 -> Product11/1
  Product11/1 -> Gain14/1
  Sign3/1 -> Product11/2
  Abs1/1 -> Math Function3/1
  Abs2/1 -> Math Function2/1
  Abs3/1 -> Math Function1/1
  Abs4/1 -> Math Function/1
  Demux/1 -> Add4/1, Gain17/1
  Constant8/1 -> Switch/3, Switch1/1
  Abs5/1 -> Switch1/3
  Switch/1 -> Product3/1, Product/1
  Gain17/1 -> Switch/2, Switch/1, Switch1/2, Abs5/1
  x/1 -> Demux/1
  Demux/2 -> Mux/1, Gain18/1
  Gain16/1 -> Add4/2
  Add4/1 -> Gain19/1
  Gain19/1 -> Add5/2
  Gain18/1 -> Add5/1
  Add5/1 -> Mux/2
  Mux/1 -> x_dot/1

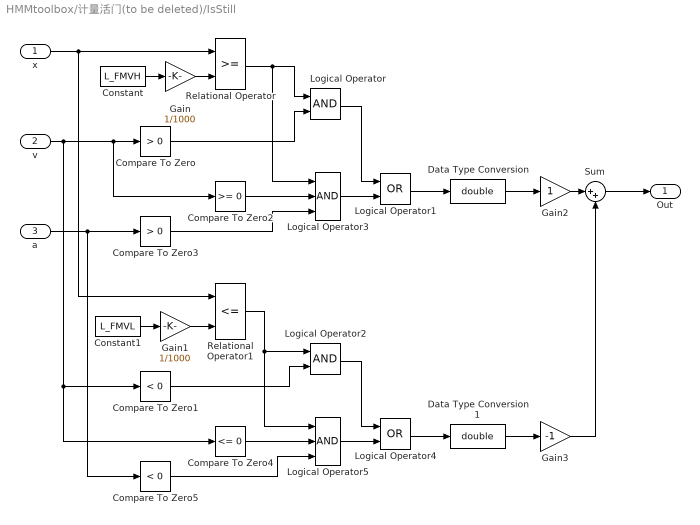
== system HMMtoolbox/计量活门(to be deleted)/IsStill ==
  x : Inport
  v : Inport  Port=2
  a : Inport  Port=3
  Compare To Zero : simulink/Logic and Bit Operations/Compare To Zero  relop=>  OutDataTypeStr=boolean  ZeroCross=off
  Compare To Zero1 : simulink/Logic and Bit Operations/Compare To Zero  relop=<  OutDataTypeStr=boolean  ZeroCross=off
  Compare To Zero2 : simulink/Logic and Bit Operations/Compare To Zero  relop=>=  OutDataTypeStr=boolean
  Compare To Zero3 : simulink/Logic and Bit Operations/Compare To Zero  relop=>  OutDataTypeStr=boolean
  Compare To Zero4 : simulink/Logic and Bit Operations/Compare To Zero  relop=<=  OutDataTypeStr=boolean  ZeroCross=off
  Compare To Zero5 : simulink/Logic and Bit Operations/Compare To Zero  relop=<  OutDataTypeStr=boolean
  Constant : Constant  Value=L_FMVH
  Constant1 : Constant  Value=L_FMVL
  Data Type Conversion : DataTypeConversion  OutDataTypeStr=double
  Data Type Conversion1 : DataTypeConversion  OutDataTypeStr=double
  Gain : Gain  Gain=1/1000
  Gain1 : Gain  Gain=1/1000
  Gain2 : Gain
  Gain3 : Gain  Gain=-1
  Logical Operator : Logic  AllPortsSameDT=off  OutDataTypeStr=boolean
  Logical Operator1 : Logic  Operator=OR  AllPortsSameDT=off  OutDataTypeStr=boolean
  Logical Operator2 : Logic  AllPortsSameDT=off  OutDataTypeStr=boolean
  Logical Operator3 : Logic  Inputs=3  AllPortsSameDT=off  OutDataTypeStr=boolean
  Logical Operator4 : Logic  Operator=OR  AllPortsSameDT=off  OutDataTypeStr=boolean
  Logical Operator5 : Logic  Inputs=3  AllPortsSameDT=off  OutDataTypeStr=boolean
  Relational Operator : RelationalOperator  OutDataTypeStr=boolean
  Relational Operator1 : RelationalOperator  Operator=<=  OutDataTypeStr=boolean  ZeroCross=off
  Sum : Sum  Inputs=|++
  Out : Outport
  wires:
  Compare To Zero5/1 -> Logical Operator5/3
  Compare To Zero4/1 -> Logical Operator5/2
  Relational Operator1/1 -> Logical Operator2/1, Logical Operator5/1
  Logical Operator4/1 -> Data Type Conversion1/1
  Logical Operator5/1 -> Logical Operator4/2
  Logical Operator2/1 -> Logical Operator4/1
  Logical Operator3/1 -> Logical Operator1/2
  Compare To Zero3/1 -> Logical Operator3/3
  a/1 -> Compare To Zero3/1, Compare To Zero5/1
  Compare To Zero2/1 -> Logical Operator3/2
  Logical Operator1/1 -> Data Type Conversion/1
  Data Type Conversion1/1 -> Gain3/1
  Data Type Conversion/1 -> Gain2/1
  Gain3/1 -> Sum/2
  Gain2/1 -> Sum/1
  Relational Operator/1 -> Logical Operator/1, Logical Operator3/1
  Constant/1 -> Gain/1
  Compare To Zero/1 -> Logical Operator/2
  Logical Operator/1 -> Logical Operator1/1
  x/1 -> Relational Operator/1, Relational Operator1/1
  Compare To Zero1/1 -> Logical Operator2/2
  v/1 -> Compare To Zero/1, Compare To Zero2/1, Compare To Zero1/1, Compare To Zero4/1
  Constant1/1 -> Gain1/1
  Gain/1 -> Relational Operator/2
  Gain1/1 -> Relational Operator1/2
  Sum/1 -> Out/1

== matlab function 泵类/ZSB/柱塞 ==
  data: P_ZSBO input double; P_ZSBI input double; base_z input double; L_ZSBHX input double; D_ZSBZS input double; RHO input double; A_ZSBZS input double; ETA_V input double; BETA_ZSBZS input double; omega input double; alpha input double; TorquePP output double; W_ZSB output double; OthrData output double; phi input double
function [ TorquePP, W_ZSB, OthrData ] = Plunger_Pump(P_ZSBO,  P_ZSBI,  base_z, L_ZSBHX, D_ZSBZS, RHO, A_ZSBZS, ETA_V,BETA_ZSBZS,omega,alpha,phi )
r=D_ZSBZS/2;
z = length( base_z );
S_max = 2 * r * tan( phi );
alpha_tab =  alpha + base_z * 2 * pi / z;
v_tab = -r * sin( alpha_tab ) * tan( phi ) * omega;
l_tab = r * cos( alpha_tab ) / cos( phi ) + L_ZSBHX * tan( phi );

p_tab = base_z;
for i = 1 : z
    if ( alpha_tab( i ) >= pi )
        alpha_tab( i ) =  alpha_tab( i ) - 2 * pi;
    end
    if ( alpha_tab( i ) < 0 )
        p_tab( i ) = P_ZSBO;
    else
        p_tab( i ) = P_ZSBI;
        v_tab( i ) = 0;
    end
end
f_tab = A_ZSBZS * p_tab / cos( phi );
m_tab = l_tab .* f_tab * 1e-6;

TorquePP = -sum( m_tab ); 

%-- Calculate q_tab and total Q --
q_tab = A_ZSBZS * ETA_V*cos(BETA_ZSBZS) * v_tab * RHO * 1e-9; 
W_ZSB = sum( q_tab );
Q2 = RHO * ETA_V *cos(BETA_ZSBZS)* A_ZSBZS * S_max * z * omega * 0.5 / pi * 1e-9;

OthrData = [ Q2, TorquePP, S_max, v_tab( z ), q_tab( z ), l_tab( z ), f_tab( z ), m_tab( z ) ];

end

== matlab function 泵类/ZSB/调节机构 ==
  data: P_ZSBO input double; TorqueFP output double; P_ZSBC input double; L_x0 input double; L_ZSBTJ input double; A_ZSBTJ input double; k input double; BETA input double; phi input double
function TorqueFP= TJ( P_ZSBO, P_ZSBC, L_x0, L_ZSBTJ, A_ZSBTJ, k, BETA, phi)

%计算活塞位置
xp = L_ZSBTJ(4)+L_ZSBTJ(1)*sin(phi+BETA)-L_ZSBTJ(5)-sqrt(L_ZSBTJ(3)*L_ZSBTJ(3)-(L_ZSBTJ(2)-L_ZSBTJ(1)*cos(phi+BETA))^2);

%计算随动活塞杆上的作用力
Pleft = P_ZSBO * 1e3;%kPa
Pright = Pleft-P_ZSBC * 1e3;%kPa
Fleft = Pleft * A_ZSBTJ(1) * 1e-6;%N
Fright = Pright * A_ZSBTJ(2) * 1e-6;%N
Fs = k * (L_x0 - xp) * 1e-3;
Fsui = Fs + Fright - Fleft;

%计算随动活塞杆力对斜盘作用力矩
delta = asin((L_ZSBTJ(2)-L_ZSBTJ(1)*cos(phi+BETA))/L_ZSBTJ(3));
TorqueFP = Fsui/cos(delta)*cos(delta-phi-BETA)*L_ZSBTJ(1)*1e-3;

end

== matlab function 泵类/ZSB/斜盘动力学方程 ==
  data: TorquePP input double; Wdot output double; TorqueFP input double; J_ZSBXP input double; W input double; KD input double
function Wdot = DL(TorquePP,TorqueFP,J_ZSBXP,W, KD) 

    Torq_Net = TorquePP + TorqueFP - W * KD;
    Wdot =  Torq_Net / J_ZSBXP;
end
